simulink model "Bio_batch_PP1"  (R2022a)
settings: Solver=ode15s  StartTime=0.0  StopTime=24.1  RelTol=1e-4  AbsTol=1e-4
values from neighbouring files (symbols this model uses):
  Ts = 0.1    [BioBatchDT.m]    (also in Executable1.m)
libraries: sharedTrackingLibrary x1
settings Model: SimulationMode=accelerator  Creator=DELL  LastModifiedBy=LADES
settings SolverCC: SolverResetMethod=Robust
settings DataIOCC: ReturnWorkspaceOutputs=off

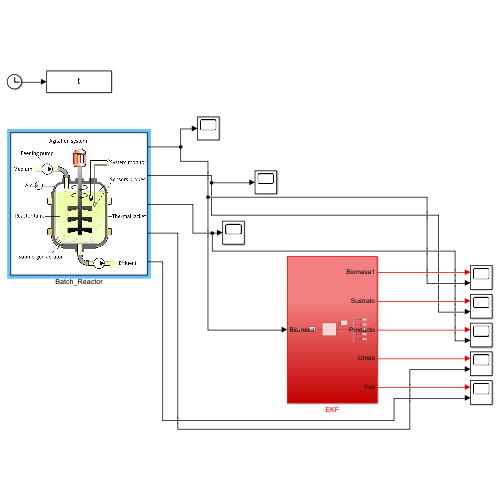
[thumbnail: Simulink's stored preview of the top-level diagram]
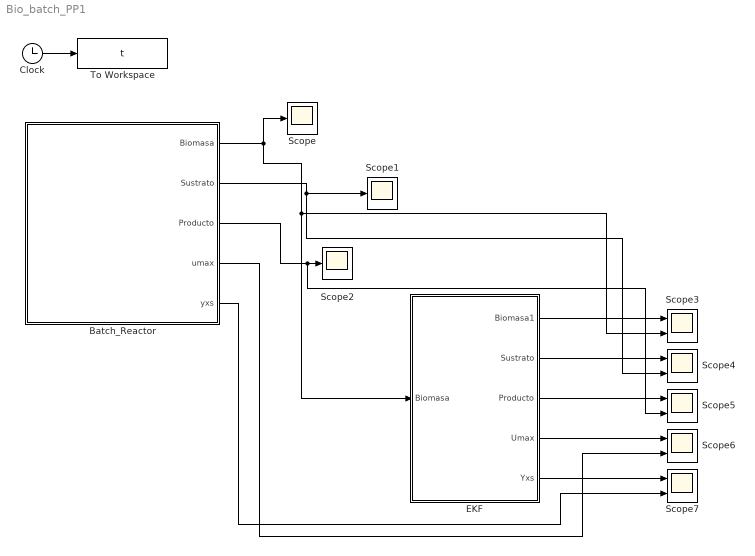
== system Bio_batch_PP1 ==
  Batch_Reactor : Subsystem
      mask Display: image('biorreactor.png'); % Use "Edit Image" on toolstrip to change.
  Clock : Clock
  EKF : Subsystem
  Scope : Scope
  Scope1 : Scope
  Scope2 : Scope
  Scope{3..7} (5 alike) : Scope  NumInputPorts=2
  To Workspace : ToWorkspace  VariableName=t  SampleTime=0.1
  wires:
  Clock/1 -> To Workspace/1
  EKF/1(Biomasa1) -> Scope3/1
  EKF/2(Sustrato) -> Scope4/1
  EKF/3(Producto) -> Scope5/1
  EKF/4(Umax) -> Scope6/1
  EKF/5(Yxs) -> Scope7/1
  Batch_Reactor/2(Sustrato) -> Scope4/2, Scope1/1
  Batch_Reactor/1(Biomasa) -> Scope/1, EKF/1(Biomasa), Scope3/2
  Batch_Reactor/3(Producto) -> Scope5/2, Scope2/1
  Batch_Reactor/4(umax) -> Scope6/2
  Batch_Reactor/5(yxs) -> Scope7/2

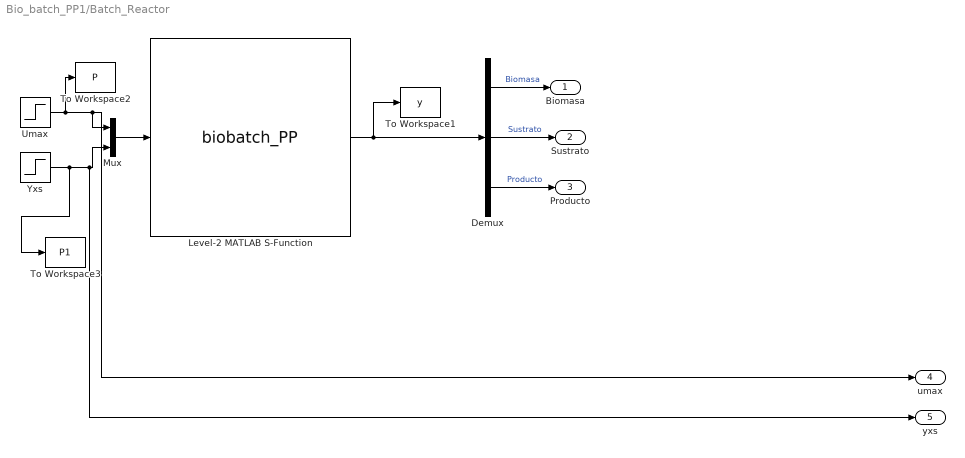
== system Bio_batch_PP1/Batch_Reactor ==
  Demux : Demux  Outputs=3
  Level-2 MATLAB S-Function : M-S-Function  FunctionName=biobatch_PP  Parameters=0.01, 20, 0
      mask Display: image('biorreactor.png'); % Use "Edit Image" on toolstrip to change.
  Mux : Mux  Inputs=2
  To Workspace1 : ToWorkspace  VariableName=y  SampleTime=0.1
  To Workspace2 : ToWorkspace  VariableName=P  SampleTime=0.1
  To Workspace3 : ToWorkspace  VariableName=P1  SampleTime=0.1
  Umax : Step  Time=24.1/2  Before=0.83  After=0.83  SampleTime=0.1
  Yxs : Step  Time=24.1/2  Before=0.8  After=0.8  SampleTime=0.1
  Biomasa : Outport
  Sustrato : Outport  Port=2
  Producto : Outport  Port=3
  umax : Outport  Port=4
  yxs : Outport  Port=5
  wires:
  Level-2 MATLAB S-Function/1 -> Demux/1, To Workspace1/1
  Mux/1 -> Level-2 MATLAB S-Function/1
  Yxs/1 -> To Workspace3/1, yxs/1, Mux/2
  Demux/2 -> Sustrato/1  "Sustrato"
  Umax/1 -> To Workspace2/1, umax/1, Mux/1
  Demux/3 -> Producto/1  "Producto"
  Demux/1 -> Biomasa/1  "Biomasa"

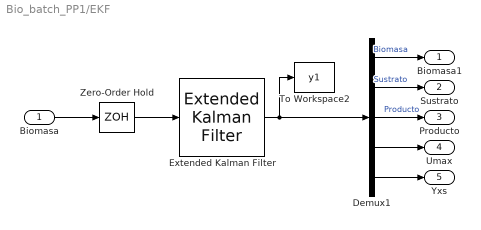
== system Bio_batch_PP1/EKF ==
  Biomasa : Inport
  Demux1 : Demux  Outputs=5
  Extended Kalman Filter : sharedTrackingLibrary/Extended Kalman Filter  StateTransitionFcn=BioBatchDT  HasStateTransitionJacobianFcn=off  HasAdditiveProcessNoise=Additive  ProcessNoise=[1e-3 1e-3 1e-3 1e2 1e2]  HasTimeVaryingProcessNoise=off  HasStateTransitionFcnExtraArgument=0  InitialState=x0  InitialStateCovariance=[1e-3 1e-3 1e-3 1e2 1e2]  MeasurementFcn1=BatchMeasFcn  HasMeasurementJacobianFcn1=off  HasMeasurementEnablePort1=off  HasAdditiveMeasurementNoise1=Additive  MeasurementNoise1=1e-3  HasTimeVaryingMeasurementNoise1=off  HasMeasurementFcnExtraArgument1=0  HasMeasurementWrapping1=off  MeasurementFcn2=myMeasurementFcn  HasMeasurementJacobianFcn2=off  HasMeasurementEnablePort2=off  HasAdditiveMeasurementNoise2=Additive  MeasurementNoise2=1  HasTimeVaryingMeasurementNoise2=off  HasMeasurementFcnExtraArgument2=0  HasMeasurementWrapping2=off  MeasurementFcn3=myMeasurementFcn  HasMeasurementJacobianFcn3=off  HasMeasurementEnablePort3=off  HasAdditiveMeasurementNoise3=Additive  MeasurementNoise3=1  HasTimeVaryingMeasurementNoise3=off  HasMeasurementFcnExtraArgument3=0  HasMeasurementWrapping3=off  MeasurementFcn4=myMeasurementFcn  HasMeasurementJacobianFcn4=off  HasMeasurementEnablePort4=off  HasAdditiveMeasurementNoise4=Additive  MeasurementNoise4=1  HasTimeVaryingMeasurementNoise4=off  HasMeasurementFcnExtraArgument4=0  HasMeasurementWrapping4=off  MeasurementFcn5=myMeasurementFcn  HasMeasurementJacobianFcn5=off  HasMeasurementEnablePort5=off  HasAdditiveMeasurementNoise5=Additive  MeasurementNoise5=1  HasTimeVaryingMeasurementNoise5=off  HasMeasurementFcnExtraArgument5=0  HasMeasurementWrapping5=off  EnableMultirate=off  StateTransitionFcnSampleTime=1  MeasurementFcn1SampleTime=1  MeasurementFcn2SampleTime=1  MeasurementFcn3SampleTime=1  MeasurementFcn4SampleTime=1  MeasurementFcn5SampleTime=1  UseCurrentEstimator=on  OutputStateCovariance=off  DataType=double  SampleTime=Ts  NumberOfMeasurements=1
      settings: SourceProductBaseCode=TF,AE,PW,CT,DR,ID,LP,NV,AR,RO,RR,UV,VE
  To Workspace2 : ToWorkspace  VariableName=y1  SampleTime=-1
  Zero-Order Hold : ZeroOrderHold  SampleTime=Ts
  Biomasa1 : Outport
  Sustrato : Outport  Port=2
  Producto : Outport  Port=3
  Umax : Outport  Port=4
  Yxs : Outport  Port=5
  wires:
  Zero-Order Hold/1 -> Extended Kalman Filter/1
  Demux1/1 -> Biomasa1/1  "Biomasa"
  Extended Kalman Filter/1 -> To Workspace2/1, Demux1/1
  Demux1/3 -> Producto/1  "Producto"
  Biomasa/1 -> Zero-Order Hold/1
  Demux1/2 -> Sustrato/1  "Sustrato"
  Demux1/4 -> Umax/1
  Demux1/5 -> Yxs/1
